simulink model "ABC_dq_park"  (R2024b)
settings: Solver=VariableStepAuto  StartTime=0.0  StopTime=10.0  RelTol=1e-3
settings Model: Creator=罗芳成  LastModifiedBy=罗芳成

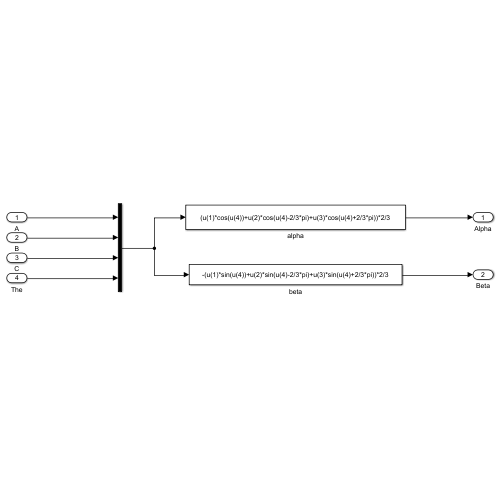
[thumbnail: Simulink's stored preview of the top-level diagram]
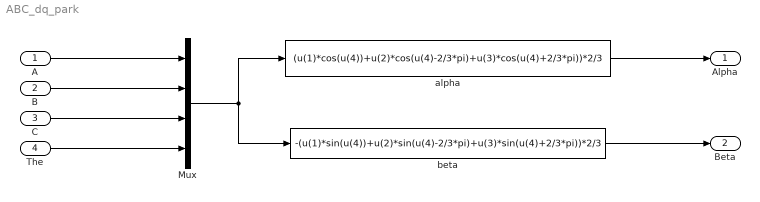
== system ABC_dq_park ==
  A : Inport
  B : Inport  Port=2
  C : Inport  Port=3
  The : Inport  Port=4
  Mux : Mux
  alpha : Fcn  Expr=(u(1)*cos(u(4))+u(2)*cos(u(4)-2/3*pi)+u(3)*cos(u(4)+2/3*pi))*2/3
  beta : Fcn  Expr=-(u(1)*sin(u(4))+u(2)*sin(u(4)-2/3*pi)+u(3)*sin(u(4)+2/3*pi))*2/3
  Alpha : Outport
  Beta : Outport  Port=2
  wires:
  A/1 -> Mux/1
  B/1 -> Mux/2
  C/1 -> Mux/3
  The/1 -> Mux/4
  Mux/1 -> beta/1, alpha/1
  alpha/1 -> Alpha/1
  beta/1 -> Beta/1
